simulink library "Lib_Piccolo"  (R2018b)
settings: Solver=VariableStepAuto  StartTime=0.0  StopTime=10.0  RelTol=1e-3
values from neighbouring files (symbols this model uses):
  AccelErrInt2Brakes = 0.15    [SimulationControlConfig16P.m]    (also in SimulationControlConfig16P_F0.m; SimulationControlConfig16P_F2.m; SimulationControlConfig16P_LEGACY.m; SimulationControlConfigTAILLESS.m = 0.2)
  AileronMax = 25    [SimulationControlConfig16P.m]    (also in SimulationControlConfig16P_F0.m; SimulationControlConfig16P_F2.m; SimulationControlConfig16P_LEGACY.m; SimulationControlConfigTAILLESS.m)
  AileronPower = 0.00268    [SimulationControlConfig16P.m]    (also in SimulationControlConfig16P_F0.m; SimulationControlConfig16P_F2.m; SimulationControlConfig16P_LEGACY.m; SimulationControlConfigTAILLESS.m = 0.002266)
  AileronSurfaceMax = 45    [SimulationControlConfig16P.m]    (also in SimulationControlConfig16P_F0.m; SimulationControlConfig16P_F2.m; SimulationControlConfig16P_LEGACY.m; SimulationControlConfigTAILLESS_CGAFT_F0.m = 25)
  AileronTrim = 0    [SimulationControlConfig16P.m]    (also in SimulationControlConfig16P_F0.m; SimulationControlConfig16P_F2.m; SimulationControlConfig16P_LEGACY.m; SimulationControlConfigTAILLESS.m)
  Alt = 1000 + TerrainHeight    [SimulationStateConfig.m]
  AltCruise_m = Alt * 0.3048    [SimulationControlConfig16P.m]    (also in SimulationControlConfig16P_F2.m; SimulationControlConfigTAILLESS.m = Alt/3.28084; SimulationControlConfigTAILLESS_CGAFT_F0.m = 640; SimulationControlConfigTAILLESS_CGFWD_F0.m = 640)
  AltitudeRate2PitchCmdIntegratorInit = 0.1    [SimulationControlPre.m]
  AltMax = 10000    [SimulationControlConfig16P.m]    (also in SimulationControlConfig16P_F0.m; SimulationControlConfig16P_F2.m; SimulationControlConfig16P_LEGACY.m; SimulationControlConfigTAILLESS.m)
  AltMaxAccel = 2.5    [SimulationControlConfig16P.m]    (also in SimulationControlConfig16P_F0.m = 2; SimulationControlConfig16P_F2.m = 2; SimulationControlConfig16P_LEGACY.m = 0.9; SimulationControlConfigTAILLESS.m = 2)
  AltMin = 0    [SimulationControlConfig16P.m]    (also in SimulationControlConfig16P_F0.m; SimulationControlConfig16P_F2.m; SimulationControlConfig16P_LEGACY.m; SimulationControlConfigTAILLESS.m)
  AltRateCmd2Pitch = 0.26    [SimulationControlConfig16P.m]    (also in SimulationControlConfig16P_F0.m = 0.35; SimulationControlConfig16P_F2.m = 0.35; SimulationControlConfig16P_LEGACY.m = 0.6; SimulationControlConfigTAILLESS.m = 0.9)
  AltRateError2Pitch = 0.34    [SimulationControlConfig16P.m]    (also in SimulationControlConfig16P_F0.m = 0.61; SimulationControlConfig16P_F2.m = 0.61; SimulationControlConfig16P_LEGACY.m = 0.4; SimulationControlConfigTAILLESS.m = 0.3)
  AltRateErrorInt2Pitch = 0.61    [SimulationControlConfig16P.m]    (also in SimulationControlConfig16P_F0.m = 0.28; SimulationControlConfig16P_F2.m = 0.28; SimulationControlConfig16P_LEGACY.m = 0.45; SimulationControlConfigTAILLESS.m = 0.15)
  AltRateLpfCutOff = 3    [SimulationControlConfig16P.m]    (also in SimulationControlConfig16P_F0.m; SimulationControlConfig16P_F2.m; SimulationControlConfig16P_LEGACY.m; SimulationControlConfigTAILLESS.m = 5)
  AutoNosegear2Rudder = 26    [SimulationControlConfig16P.m]    (also in SimulationControlConfig16P_F0.m; SimulationControlConfig16P_F2.m; SimulationControlConfig16P_LEGACY.m; SimulationControlConfigTAILLESS.m = 25.2)
  b = 5.54    [SimulationControlConfig16P.m]    (also in SimulationControlConfig16P_F0.m; SimulationControlConfig16P_F2.m; SimulationControlConfig16P_LEGACY.m; SimulationControlConfigTAILLESS.m = 2.37)
  Bank2AileronIntegratorInit = 0    [SimulationControlPre.m]
  BankMax_User = BankMax_User/180*pi    (= 0.610865238198)    [SimulationControlConfig16P.m]    (also in SimulationControlConfig16P_F0.m = 0.523598775598; SimulationControlConfig16P_F2.m = 0.523598775598; SimulationControlConfig16P_LEGACY.m = 0.523598775598; SimulationControlConfigTAILLESS.m = 0.558505360638)
  baseLegFlaps = 20    [SimulationControlConfig16P.m]    (also in SimulationControlConfig16P_F0.m; SimulationControlConfig16P_F2.m = 15; SimulationControlConfig16P_LEGACY.m = 0; SimulationControlConfigTAILLESS.m = 0)
  C = GeneticOpt.C    [SimulationCostFunction.m]
  c = Sw/b    (= 0.841696750903)    [SimulationControlConfig16P.m]    (also in SimulationControlConfig16P_F0.m; SimulationControlConfig16P_F2.m; SimulationControlConfig16P_LEGACY.m; SimulationControlConfigTAILLESS.m = 0.354008438819)
  cell2WheelFactorMG = 5.98    [SimulationSensorConfig16P_LEGACY.m]
  cell2WheelFactorNG = 1    [SimulationSensorConfig16P_LEGACY.m]
  cellSatMaxMG = 15000    [SimulationSensorConfig16P.m]    (also in SimulationSensorConfig16P_LEGACY.m; SimulationSensorConfigTAILLESS7P.m; SimulationSensorConfigUTAIL7P.m)
  cellSatMaxNG = 1000    [SimulationSensorConfig16P.m]    (also in SimulationSensorConfig16P_LEGACY.m; SimulationSensorConfigTAILLESS7P.m; SimulationSensorConfigUTAIL7P.m)
  cellSatMinMG = -15000    [SimulationSensorConfig16P.m]    (also in SimulationSensorConfig16P_LEGACY.m; SimulationSensorConfigTAILLESS7P.m; SimulationSensorConfigUTAIL7P.m)
  cellSatMinNG = -1000    [SimulationSensorConfig16P.m]    (also in SimulationSensorConfig16P_LEGACY.m; SimulationSensorConfigTAILLESS7P.m; SimulationSensorConfigUTAIL7P.m)
  CL_Limit = CL_Max    (= 0.54)    [SimulationControlConfig16P.m]    (also in SimulationControlConfig16P_F0.m; SimulationControlConfig16P_F2.m = 0.638; SimulationControlConfig16P_LEGACY.m; SimulationControlConfigTAILLESS.m = 0.525)
  CL_Max = 0.54    [SimulationControlConfig16P.m]    (also in SimulationControlConfig16P_F0.m; SimulationControlConfig16P_F2.m = 0.638; SimulationControlConfig16P_LEGACY.m; SimulationControlConfigTAILLESS.m = 0.525)
  CL_Max_Nom = 0.465    [SimulationControlConfig16P.m]    (also in SimulationControlConfig16P_F0.m; SimulationControlConfig16P_F2.m = 0.563; SimulationControlConfig16P_LEGACY.m; SimulationControlConfigTAILLESS.m = 0.39)
  CL_Min = 0    [SimulationControlConfig16P.m]    (also in SimulationControlConfig16P_F0.m; SimulationControlConfig16P_F2.m; SimulationControlConfig16P_LEGACY.m; SimulationControlConfigTAILLESS.m)
  ClimbMaxFraction = 0.35    [SimulationControlConfig16P.m]    (also in SimulationControlConfig16P_F0.m = 0.17; SimulationControlConfig16P_F2.m = 0.17; SimulationControlConfig16P_LEGACY.m = 0.24; SimulationControlConfigTAILLESS.m = 0.21)
  ClimboutMaxBank = 7.0    (= 7)    [SimulationControlConfig16P.m]    (also in SimulationControlConfig16P_F0.m; SimulationControlConfig16P_F2.m; SimulationControlConfig16P_LEGACY.m; SimulationControlConfigTAILLESS.m = 5)
  ClimboutTimer = 7.0    (= 7)    [SimulationControlConfig16P.m]    (also in SimulationControlConfig16P_F0.m; SimulationControlConfig16P_F2.m; SimulationControlConfig16P_LEGACY.m; SimulationControlConfigTAILLESS.m)
  dCl_per_dFlap = 0.005581818    [SimulationControlConfig16P.m]    (also in SimulationControlConfig16P_F0.m = 0; SimulationControlConfig16P_F2.m = 0.0065; SimulationControlConfig16P_LEGACY.m = 0; SimulationControlConfigTAILLESS.m = 0)
  DecelerationCmd = 3.1    [SimulationControlConfig16P.m]    (also in SimulationControlConfig16P_F0.m; SimulationControlConfig16P_F2.m; SimulationControlConfig16P_LEGACY.m; SimulationControlConfigTAILLESS.m = 0.1)
  DeRotateLogicEndTimer = abs((NoseDownLimit_Deg-1)/DeRotateRamp_Dps)    [SimulationControlConfig16P.m]    (also in SimulationControlConfig16P_F0.m; SimulationControlConfig16P_F2.m; SimulationControlConfig16P_LEGACY.m; SimulationControlConfigTAILLESS.m)
  DeRotateLogicHoldNoseUpTimer = 0.1    [SimulationControlConfig16P.m]    (also in SimulationControlConfig16P_F0.m; SimulationControlConfig16P_F2.m; SimulationControlConfig16P_LEGACY.m; SimulationControlConfigTAILLESS.m)
  DeRotateLogicTimerTimeout = 2    [SimulationControlConfig16P.m]    (also in SimulationControlConfig16P_F0.m; SimulationControlConfig16P_F2.m; SimulationControlConfig16P_LEGACY.m; SimulationControlConfigTAILLESS.m)
  DeRotateLowerCmdSaturation = 0    [SimulationControlConfig16P.m]    (also in SimulationControlConfig16P_F0.m; SimulationControlConfig16P_F2.m; SimulationControlConfig16P_LEGACY.m; SimulationControlConfigTAILLESS.m)
  DeRotateRamp_Dps = 3    [SimulationControlConfig16P.m]    (also in SimulationControlConfig16P_F0.m; SimulationControlConfig16P_F2.m; SimulationControlConfig16P_LEGACY.m; SimulationControlConfigTAILLESS.m = 8)
  DeRotateUpperCmdSaturation = 7    [SimulationControlConfig16P.m]    (also in SimulationControlConfig16P_F0.m; SimulationControlConfig16P_F2.m; SimulationControlConfig16P_LEGACY.m; SimulationControlConfigTAILLESS.m)
  DescentMaxFraction = 0.22    [SimulationControlConfig16P.m]    (also in SimulationControlConfig16P_F0.m = 0.2; SimulationControlConfig16P_F2.m = 0.2; SimulationControlConfig16P_LEGACY.m = 0.2; SimulationControlConfigTAILLESS.m = 0.17)
  DesktopSimTerrainOffset_m = 0.406    [SimulationAircraftConfig.m]
  downwindFlaps = 0    [SimulationControlConfig16P.m]    (also in SimulationControlConfig16P_F0.m; SimulationControlConfig16P_F2.m = 15; SimulationControlConfig16P_LEGACY.m; SimulationControlConfigTAILLESS.m)
  downwindSplitAil = 0    [SimulationControlConfig16P_F2.m]
  DP_init = 0.5*1.225*V_init^2    [SimulationControlConfig16P.m]    (also in SimulationControlConfig16P_F0.m; SimulationControlConfig16P_F2.m; SimulationControlConfig16P_LEGACY.m; SimulationControlConfigTAILLESS.m)
  dscNoiseMG = 1    [SimulationSensorConfig16P_LEGACY.m]
  dscNoiseNG = 0.25    [SimulationSensorConfig16P_LEGACY.m]
  DSCnumBits = 24    [SimulationSensorConfig16P.m]    (also in SimulationSensorConfig16P_LEGACY.m; SimulationSensorConfigTAILLESS7P.m; SimulationSensorConfigUTAIL7P.m)
  DSCRangeMaxMG = 15000    [SimulationSensorConfig16P.m]    (also in SimulationSensorConfig16P_LEGACY.m; SimulationSensorConfigTAILLESS7P.m; SimulationSensorConfigUTAIL7P.m)
  DSCRangeMaxNG = 1000    [SimulationSensorConfig16P.m]    (also in SimulationSensorConfig16P_LEGACY.m; SimulationSensorConfigTAILLESS7P.m; SimulationSensorConfigUTAIL7P.m)
  DSCRangeMinMG = -15000    [SimulationSensorConfig16P.m]    (also in SimulationSensorConfig16P_LEGACY.m; SimulationSensorConfigTAILLESS7P.m; SimulationSensorConfigUTAIL7P.m)
  DSCRangeMinNG = -1000    [SimulationSensorConfig16P.m]    (also in SimulationSensorConfig16P_LEGACY.m; SimulationSensorConfigTAILLESS7P.m; SimulationSensorConfigUTAIL7P.m)
  dt = DLLSim.dt    [SimulationTimeStep.m]    (also in SimulationTrim.m = 0.02)
  EarlyTouchdownThreshold = 3.0    (= 3)    [SimulationControlConfig16P.m]    (also in SimulationControlConfig16P_F0.m; SimulationControlConfig16P_F2.m; SimulationControlConfig16P_LEGACY.m; SimulationControlConfigTAILLESS.m)
  ElevatorDeflectionRate = 15    [SimulationControlConfig16P.m]    (also in SimulationControlConfig16P_F0.m; SimulationControlConfig16P_F2.m; SimulationControlConfig16P_LEGACY.m = 12; SimulationControlConfigTAILLESS.m = 5)
  ElevatorMax = 25    [SimulationControlConfig16P.m]    (also in SimulationControlConfig16P_F0.m; SimulationControlConfig16P_F2.m; SimulationControlConfig16P_LEGACY.m; SimulationControlConfigTAILLESS.m)
  ElevatorPower = -0.002209    [SimulationControlConfig16P.m]    (also in SimulationControlConfig16P_F0.m; SimulationControlConfig16P_F2.m; SimulationControlConfig16P_LEGACY.m; SimulationControlConfigTAILLESS.m = -0.002668)
  ElevatorTrim = -3.5    [SimulationControlConfig16P.m]    (also in SimulationControlConfig16P_F0.m; SimulationControlConfig16P_F2.m; SimulationControlConfig16P_LEGACY.m; SimulationControlConfigTAILLESS.m = -3)
  elevonBias = 0    [SimulationControlConfig16P.m]    (also in SimulationControlConfig16P_F0.m; SimulationControlConfig16P_F2.m; SimulationControlConfig16P_LEGACY.m; SimulationControlConfigTAILLESS.m)
  Enable_TAS_Protection = 0    [SimulationControlConfig16P.m]    (also in SimulationControlConfig16P_F0.m; SimulationControlConfig16P_F2.m; SimulationControlConfig16P_LEGACY.m; SimulationControlConfigTAILLESS.m)
  EnableCrossTrackAbort = 1    [SimulationControlConfig16P.m]    (also in SimulationControlConfigTAILLESS.m; SimulationControlConfigTAILLESS_CGAFT_F0.m; SimulationControlConfigTAILLESS_CGFWD_F0.m; SimulationControlConfigTAILLESS_CGFWD_F2.m)
  EnergyBandwidth = 0.04    [SimulationControlConfig16P.m]    (also in SimulationControlConfig16P_F0.m = 0.03; SimulationControlConfig16P_F2.m = 0.03; SimulationControlConfig16P_LEGACY.m = 0.02; SimulationControlConfigTAILLESS.m = 0.06)
  EngineLhFuelCut = 0    [SimulationAircraftConfig.m]
  EngineRhFuelCut = 0    [SimulationAircraftConfig.m]
  FastThrottleRate = 0.075    [SimulationControlConfig16P.m]    (also in SimulationControlConfig16P_F0.m = 0.05; SimulationControlConfig16P_F2.m = 0.05; SimulationControlConfig16P_LEGACY.m = 0.05; SimulationControlConfigTAILLESS.m = 0.1)
  FilterWarmUpTime = 2    [SimulationSensorConfig16P.m]    (also in SimulationSensorConfig16P_LEGACY.m; SimulationSensorConfigTAILLESS7P.m; SimulationSensorConfigUTAIL7P.m)
  finalApproachFlaps = 20    [SimulationControlConfig16P.m]    (also in SimulationControlConfig16P_F0.m; SimulationControlConfig16P_F2.m = 15; SimulationControlConfig16P_LEGACY.m = 0; SimulationControlConfigTAILLESS.m = 0)
  finalApproachSplitAil = 20    [SimulationControlConfig16P_F2.m]
  FinalDescentSlope_Deg = testPlans(testIndx).descentSlope    [SimulationControlConfig16P.m]    (also in SimulationControlConfig16P_F0.m; SimulationControlConfig16P_F2.m; SimulationControlConfig16P_LEGACY.m; SimulationControlConfigTAILLESS.m)
  flapMax = 0    [SimulationControlConfig16P.m]    (also in SimulationControlConfig16P_F0.m = 35; SimulationControlConfig16P_F2.m = 33; SimulationControlConfig16P_LEGACY.m; SimulationControlConfigTAILLESS.m)
  flapRate = 7.5    [SimulationControlConfig16P.m]    (also in SimulationControlConfig16P_F0.m; SimulationControlConfig16P_F2.m; SimulationControlConfig16P_LEGACY.m; SimulationControlConfigTAILLESS.m = 6.6)
  FlareHeight = 5    [SimulationControlConfig16P.m]    (also in SimulationControlConfig16P_F0.m; SimulationControlConfig16P_F2.m; SimulationControlConfig16P_LEGACY.m = 4.8; SimulationControlConfigTAILLESS.m = 2.75)
  FlareVerticalRate_mps = -0.4    [SimulationControlConfig16P.m]    (also in SimulationControlConfig16P_F0.m; SimulationControlConfig16P_F2.m; SimulationControlConfig16P_LEGACY.m = -0.5; SimulationControlConfigTAILLESS.m = -0.15)
  Fp_Aileron = 0.55*2*pi*RollRateLpfCutoff*dt    [SimulationControlConfig16P.m]    (also in SimulationControlConfig16P_F0.m; SimulationControlConfig16P_F2.m; SimulationControlConfig16P_LEGACY.m; SimulationControlConfigTAILLESS.m)
  Fp_Alt = 2*pi*0.55*AltBandwidth    (= 0.622035345411)    [SimulationControlConfig16P.m]    (also in SimulationControlConfig16P_F0.m; SimulationControlConfig16P_F2.m; SimulationControlConfig16P_LEGACY.m = 0.099; SimulationControlConfigTAILLESS.m = 0.207345115137)
  Fp_AltRate = 0.55*2*pi*AltRateLpfCutOff*dt    [SimulationControlConfig16P.m]    (also in SimulationControlConfig16P_F0.m; SimulationControlConfig16P_F2.m; SimulationControlConfig16P_LEGACY.m; SimulationControlConfigTAILLESS.m)
  Fp_Elevator = 0.55*2*pi*PitchRateLpfCutoff*dt    [SimulationControlConfig16P.m]    (also in SimulationControlConfig16P_F0.m; SimulationControlConfig16P_F2.m; SimulationControlConfig16P_LEGACY.m; SimulationControlConfigTAILLESS.m)
  Fp_Energy = 0.55*2*pi*EnergyBandwidth    (= 0.138230076758)    [SimulationControlConfig16P.m]    (also in SimulationControlConfig16P_F0.m = 0.103672557568; SimulationControlConfig16P_F2.m = 0.103672557568; SimulationControlConfig16P_LEGACY.m = 0.069115038379; SimulationControlConfigTAILLESS.m = 0.207345115137)
  Fp_Energy2 = 0.55*2*pi*EnergyBandwidth*dt    [SimulationControlConfig16P.m]    (also in SimulationControlConfig16P_F0.m; SimulationControlConfig16P_F2.m; SimulationControlConfig16P_LEGACY.m; SimulationControlConfigTAILLESS.m)
  Fp_Pitch = 0.55*2*pi*PitchBandwidth    (= 2.45358386245)    [SimulationControlConfig16P.m]    (also in SimulationControlConfig16P_F0.m; SimulationControlConfig16P_F2.m = 1.72787595947; SimulationControlConfig16P_LEGACY.m = 3.11017672705; SimulationControlConfigTAILLESS.m = 1.55508836353)
  Fp_Pitch_2 = 0.55*2*pi*PitchBandwidth*dt    [SimulationControlConfig16P.m]    (also in SimulationControlConfig16P_F0.m; SimulationControlConfig16P_F2.m; SimulationControlConfig16P_LEGACY.m; SimulationControlConfigTAILLESS.m)
  Fp_Roll = RollBandwidth^2    (= 1.69)    [SimulationControlConfig16P.m]    (also in SimulationControlConfig16P_F0.m = 1.44; SimulationControlConfig16P_F2.m = 1.44; SimulationControlConfig16P_LEGACY.m = 1.44; SimulationControlConfigTAILLESS.m = 1.21)
  Fp_Rudder = 0.55*2*pi*YawRateLpfCutoff*dt    [SimulationControlConfig16P.m]    (also in SimulationControlConfig16P_F0.m; SimulationControlConfig16P_F2.m; SimulationControlConfig16P_LEGACY.m; SimulationControlConfigTAILLESS.m)
  Fp_TAS = 0.55*2*pi*TASBandwidth    (= 0.103672557568)    [SimulationControlConfig16P.m]    (also in SimulationControlConfig16P_F0.m; SimulationControlConfig16P_F2.m; SimulationControlConfig16P_LEGACY.m; SimulationControlConfigTAILLESS.m = 0.172787595947)
  Fp_TAS_Filter = 2*pi*TasLpfCutoff*dt    [SimulationControlConfig16P.m]    (also in SimulationControlConfig16P_F0.m; SimulationControlConfig16P_F2.m; SimulationControlConfig16P_LEGACY.m; SimulationControlConfigTAILLESS.m)
  Fp_Turn = 0.55*2*pi*TurnErrLPFcutoff    (= 0.172787595947)    [SimulationControlConfig16P.m]    (also in SimulationControlConfig16P_F0.m = 0.0345575191895; SimulationControlConfig16P_F2.m = 0.0345575191895; SimulationControlConfig16P_LEGACY.m = 0.0345575191895; SimulationControlConfigTAILLESS.m)
  Fp_TurnDerr = 0.55*2*pi*TurnDerivativeLPFcutoff    (= 0.172787595947)    [SimulationControlConfig16P.m]    (also in SimulationControlConfig16P_F0.m = 0.0345575191895; SimulationControlConfig16P_F2.m = 0.0345575191895; SimulationControlConfig16P_LEGACY.m = 0.0345575191895; SimulationControlConfigTAILLESS.m)
  FTV = 3    [SimulationAircraftConfig.m]
  ftvStaticPositionError = 1/1.18    (= 0.847457627119)    [SimulationSensorConfig16P.m]    (also in SimulationSensorConfig16P_LEGACY.m; SimulationSensorConfigTAILLESS7P.m = 1; SimulationSensorConfigUTAIL7P.m = 1)
  g = 9.81    [SimulationStateConfig.m]
  goAroundSplitAil = 0    [SimulationControlConfig16P_F2.m]
  GustSpd_Kts = testPlans(testIndx).gustSpd    [SimulationStateConfig.m]
  GustTriggerVal = testPlans(testIndx).gustTriggerVal    [SimulationStateConfig.m]
  HeadingErr2TurnRate = 0.5    [SimulationControlConfig16P.m]    (also in SimulationControlConfig16P_F0.m; SimulationControlConfig16P_F2.m; SimulationControlConfig16P_LEGACY.m; SimulationControlConfigTAILLESS.m)
  HeadingErrDer2TurnRate = 0.3    [SimulationControlConfig16P.m]    (also in SimulationControlConfig16P_F0.m; SimulationControlConfig16P_F2.m; SimulationControlConfig16P_LEGACY.m; SimulationControlConfigTAILLESS.m)
  IASbounce = IASstall*0.8    [SimulationControlPre.m]
  IAScruiseCMD = sqrt(2*m*9.81/(1.225*Sw*CL_cruise))    [SimulationControlConfig16P.m]    (also in SimulationControlConfig16P_F0.m; SimulationControlConfig16P_F2.m; SimulationControlConfig16P_LEGACY.m; SimulationControlConfigTAILLESS.m)
  IASfinalCMD = 1.12 * IASmin    [SimulationControlConfig16P.m]    (also in SimulationControlConfig16P_F0.m = 1.14 * IASmin; SimulationControlConfig16P_F2.m = 1.10 * IASmin; SimulationControlConfig16P_LEGACY.m = 1.10 * IASmin; SimulationControlConfigTAILLESS.m = 1.14 * IASmin)
  IASflareCMD = IASstall    [SimulationControlConfig16P.m]    (also in SimulationControlConfig16P_F0.m; SimulationControlConfig16P_F2.m; SimulationControlConfig16P_LEGACY.m; SimulationControlConfigTAILLESS.m)
  IASmax = 64    [SimulationControlConfig16P.m]    (also in SimulationControlConfig16P_F0.m = 46; SimulationControlConfig16P_F2.m = 52; SimulationControlConfig16P_LEGACY.m = 46; SimulationControlConfigTAILLESS.m = 38.9)
  IASmin = sqrt(2*m*9.81/(1.225*Sw*0.9*CL_Max_Nom))    [SimulationControlConfig16P.m]    (also in SimulationControlConfig16P_F0.m; SimulationControlConfig16P_F2.m; SimulationControlConfig16P_LEGACY.m; SimulationControlConfigTAILLESS.m)
  IASshortCMD = IASstall    [SimulationControlConfig16P.m]    (also in SimulationControlConfig16P_F0.m; SimulationControlConfig16P_F2.m; SimulationControlConfig16P_LEGACY.m; SimulationControlConfigTAILLESS.m)
  IASstall = sqrt(2*m*9.81/(1.225*Sw*CL_Max))    [SimulationControlConfig16P.m]    (also in SimulationControlConfig16P_F0.m; SimulationControlConfig16P_F2.m; SimulationControlConfig16P_LEGACY.m; SimulationControlConfigTAILLESS.m)
  inFlight = 1    [SimulationControlConfig16P.m]    (also in SimulationControlConfigTAILLESS.m; SimulationControlConfigTAILLESS_CGAFT_F0.m; SimulationControlConfigTAILLESS_CGFWD_F0.m; SimulationControlConfigTAILLESS_CGFWD_F2.m)
  JetCatOffset = 5    [SimulationControlConfig16P.m]    (also in SimulationControlConfig16P_F0.m; SimulationControlConfig16P_F2.m; SimulationControlConfig16P_LEGACY.m)
  LaunchRollingElevator = -1.5    [SimulationControlConfig16P.m]    (also in SimulationControlConfig16P_F0.m; SimulationControlConfig16P_F2.m = 1.25; SimulationControlConfig16P_LEGACY.m; SimulationControlConfigTAILLESS.m = 1)
  ldg_NosegearMax = 10    [SimulationControlConfig16P.m]    (also in SimulationControlConfig16P_F0.m; SimulationControlConfig16P_F2.m; SimulationControlConfig16P_LEGACY.m; SimulationControlConfigTAILLESS.m)
  ldg_TrackVyErrInt2Nosegear = 0.1250    (= 0.125)    [SimulationControlConfig16P.m]    (also in SimulationControlConfig16P_F0.m; SimulationControlConfig16P_F2.m; SimulationControlConfig16P_LEGACY.m; SimulationControlConfigTAILLESS.m = 0.00714285714286)
  ldg_TrackVyErrPro2Nosegear = 0.35    [SimulationControlConfig16P.m]    (also in SimulationControlConfig16P_F0.m; SimulationControlConfig16P_F2.m; SimulationControlConfig16P_LEGACY.m; SimulationControlConfigTAILLESS.m = 0.0546666666667)
  ldg_TrackY2Vy = 0.07    [SimulationControlConfig16P.m]    (also in SimulationControlConfig16P_F0.m; SimulationControlConfig16P_F2.m; SimulationControlConfig16P_LEGACY.m; SimulationControlConfigTAILLESS.m = 0.17)
  ldg_Vy2NosegearScalingPower = 1.075    [SimulationControlConfig16P.m]    (also in SimulationControlConfig16P_F0.m; SimulationControlConfig16P_F2.m; SimulationControlConfig16P_LEGACY.m; SimulationControlConfigTAILLESS.m = 0.6)
  ldg_Y2VyScalingPower = 0.175    [SimulationControlConfig16P.m]    (also in SimulationControlConfig16P_F0.m; SimulationControlConfig16P_F2.m; SimulationControlConfig16P_LEGACY.m; SimulationControlConfigTAILLESS.m = 0)
  ldg_YawRate2Nosegear = 0.175    [SimulationControlConfig16P.m]    (also in SimulationControlConfig16P_F0.m; SimulationControlConfig16P_F2.m; SimulationControlConfig16P_LEGACY.m; SimulationControlConfigTAILLESS.m = 0.065)
  LiftSlope = 0.064285    [SimulationControlConfig16P.m]    (also in SimulationControlConfig16P_F0.m; SimulationControlConfig16P_F2.m; SimulationControlConfig16P_LEGACY.m; SimulationControlConfigTAILLESS.m = 0.058631)
  LPFaileronInit = 0    [SimulationControlPre.m]
  LPFclestInit = 0    [SimulationControlPre.m]
  LPFenergyFFInit = 0    [SimulationControlPre.m]
  ... (+122 more)
undefined symbols (not defined in the file or in its folder): abortFlag, alphaHPF, apmDelay, BRWNOUT, CRAWOR, CRAWUR, DiscIntNeverNeededParam, DLLSim, DLLSimStep, ECOMOR, ECOMUR, Fp_Tas, GustTrigger_HeightAgl_m, IPSTAT, LCINTEG, Ldg_Persist_Time, LOWER_FLAGS, MSG_ENABLE, NoiseStd, OLDVAL, OVERRIDE_ENABLE, OVERRIDE_VALUE, REBOOT, reversionEnable, revIASMax, revIASMin, revPitchMax, revPitchMin, revPitchRateMax, revRollMax, revRollRateMax, SAMPLE, SCALON, SensorModel, sigbuilder_block, Sim_Vx, Sim_Vy, Sim_Vz, Sim_Xpos, Sim_Ypos, Sim_Zpos, SYSOR, SYSUR, TARE, TEMPOR, TEMPUR, testIndx, testPlan, testPlans, Trim_piccoloInCmd, Trim_REFSI_FD_IN_nmodeCgShifterCmd_Flag, Trim_REFSI_FD_IN_nmodeCgShifterCmd_Ft, Trim_REFSI_FD_IN_nmodeCgShifterCmdType, Trim_REFSI_FD_IN_nmodeCgShifterNRCActive, Trim_REFSI_FD_IN_nmodeFlapLhIBCmd_Deg, Trim_REFSI_FD_IN_nmodeFlapLhOBCmd_Deg, Trim_REFSI_FD_IN_nmodeFlapRhIBCmd_Deg, Trim_REFSI_FD_IN_nmodeFlapRhOBCmd_Deg, Trim_REFSI_FD_IN_nmodeSlatLhCmd_Deg ... (+11)
libraries: simulink x1237, $bdroot x179, aerolibconvert2 x63, dspswit3 x25, aerolibatmos2 x5, simulink_extras x4, dsparch4 x2, Lib_Piccolo_Alt x2, eeGeneralControl x1, dspindex x1
(part 54 of 74)

== system Lib_Piccolo/Ground Detection Systems/WoW Wrapper/Variant Subsystem/Load Cell WoW Model 20/WOW Module/T//O Configuration ==
  note: Unlike when landing our persistance and latching is inverted relative to Weight Off both gears.
      |
      | Protection against WOW Failure. In the Event of a Sensor Failure and AC lift's off, NZ threshold overides WOW signal.
  WOW_Filt : Inport
  DSC_Fail : Inport  Port=2
  AND : Logic  IconShape=distinctive  AllPortsSameDT=off  OutDataTypeStr=boolean
  Bus Selector : BusSelector  OutputSignals=WOW_Filt_NG_N,WOW_Filt_MGL_N,WOW_Filt_MGR_N
  Bus Selector1 : BusSelector  OutputSignals=MGR_DSC_FAIL,MGL_DSC_FAIL
  Compare To Constant1 : simulink/Logic and Bit Operations/Compare To Constant  relop=<  const=SensorModel.WOW.Cell.TO_loadThreshold_N  OutDataTypeStr=uint8
  Compare To Constant2 : simulink/Logic and Bit Operations/Compare To Constant  relop=<  const=SensorModel.WOW.Cell.TO_loadThreshold_N  OutDataTypeStr=uint8
  Input Selection (Failure Handling) : $bdroot/Ground Detection Systems/WoW Wrapper/Variant Subsystem/Load Cell WoW Model 20/WOW Module/Landing Configuration/Input Selection (Failure Handling)  SystemSampleTime=-1
  Latch : Subsystem
  Latch Timer : Subsystem  mask{period=SensorModel.WOW.Cell.TO_latchTime_s}
      mask prompts: period "Period [s]"
  NOT : Logic  Operator=NOT  IconShape=distinctive  AllPortsSameDT=off  OutDataTypeStr=boolean
  NOT2 : Logic  Operator=NOT  IconShape=distinctive  AllPortsSameDT=off  OutDataTypeStr=boolean
  Persistance Timer : Subsystem  mask{period=SensorModel.WOW.Cell.TO_persistanceTime_s}
      mask prompts: period "Period [s]"
  Terminator : Terminator
  Unit Delay : UnitDelay  SampleTime=-1
  ContactBool : Outport
  Takeoff_Fail_L : Outport  Port=2
  Takeoff_Fail_R : Outport  Port=3
  wires:
  NOT2/1 -> ContactBool/1
  Persistance Timer/1(Expired) -> Latch/1(D)
  Compare To Constant2/1 -> AND/1
  Latch Timer/1(Expired) -> NOT/1
  Unit Delay/1 -> Latch Timer/1(Enable/!Rst)
  Compare To Constant1/1 -> AND/2
  AND/1 -> Persistance Timer/1(Enable/!Rst)
  Latch/1(Q_Latched) -> NOT2/1, Unit Delay/1  "ContactBool"
  NOT/1 -> Latch/2(Enable/!Rst)
  WOW_Filt/1 -> Bus Selector/1
  Bus Selector/1 -> Terminator/1  "<WOW_Filt_NG_N>"
  Bus Selector/2 -> Input Selection (Failure Handling)/1  "<WOW_Filt_MGL_N>"
  Bus Selector/3 -> Input Selection (Failure Handling)/2  "<WOW_Filt_MGR_N>"
  DSC_Fail/1 -> Bus Selector1/1
  Bus Selector1/1 -> Input Selection (Failure Handling)/3  "<MGR_DSC_FAIL>"
  Bus Selector1/2 -> Input Selection (Failure Handling)/4  "<MGL_DSC_FAIL>"
  Input Selection (Failure Handling)/1 -> Compare To Constant2/1  "InputL"
  Input Selection (Failure Handling)/2 -> Compare To Constant1/1  "InputR"
  Input Selection (Failure Handling)/3 -> Takeoff_Fail_L/1
  Input Selection (Failure Handling)/4 -> Takeoff_Fail_R/1

== system Lib_Piccolo/Ground Detection Systems/WoW Wrapper/Variant Subsystem/Load Cell WoW Model 20/WOW Module/Tare ==
  note: Use DSC health information to select tare value.
      |
      | If DSC is failed, use previous tare value (don't update).
      |
      | Else, sample LPF for that channel and update tare value.
  WOW_Bias_Filt_N : Inport
  DSC_Fail : Inport  Port=2
  Tare_In : Inport  Port=3
  Trigger : TriggerPort  VariantControl=Variant  PortDimensions=1
  Bus Selector : BusSelector  OutputSignals=Bias_NG_N,Bias_MGL_N,Bias_MGR_N
  Bus Selector1 : BusSelector  OutputSignals=NG_DSC_FAIL,MGL_DSC_FAIL,MGR_DSC_FAIL
  Bus Selector2 : BusSelector  OutputSignals=NG_TARE_N,MGL_TARE_N,MGR_TARE_N
  Switch : Switch  Criteria=u2 > Threshold  Threshold=0.5
  Switch1 : Switch  Criteria=u2 > Threshold  Threshold=0.5
  Switch2 : Switch  Criteria=u2 > Threshold  Threshold=0.5
  NG_TARE_N : Outport  OutDataTypeStr=single
  MGL_TARE_N : Outport  Port=2  OutDataTypeStr=single
  MGR_TARE_N : Outport  Port=3  OutDataTypeStr=single
  wires:
  WOW_Bias_Filt_N/1 -> Bus Selector/1
  Bus Selector/1 -> [Bias_NG_N]  "<Bias_NG_N>"
  Bus Selector/2 -> [Bias_MGL_N]  "<Bias_MGL_N>"
  Bus Selector/3 -> [Bias_MGR_N]  "<Bias_MGR_N>"
  DSC_Fail/1 -> Bus Selector1/1
  Bus Selector1/3 -> Switch2/2  "<MGR_DSC_FAIL>"
  Bus Selector1/2 -> Switch1/2  "<MGL_DSC_FAIL>"
  Bus Selector1/1 -> Switch/2  "<NG_DSC_FAIL>"
  Tare_In/1 -> Bus Selector2/1
  Bus Selector2/1 -> [NG_TARE]  "<NG_TARE_N>"
  Bus Selector2/2 -> [MGL_TARE]  "<MGL_TARE_N>"
  Bus Selector2/3 -> [MGR_TARE]  "<MGR_TARE_N>"
  [NG_TARE] -> Switch/1
  Switch/1 -> NG_TARE_N/1
  [Bias_NG_N] -> Switch/3
  Switch1/1 -> MGL_TARE_N/1
  [Bias_MGL_N] -> Switch1/3
  [MGL_TARE] -> Switch1/1
  [MGR_TARE] -> Switch2/1
  [Bias_MGR_N] -> Switch2/3
  Switch2/1 -> MGR_TARE_N/1

== system Lib_Piccolo/Ground Detection Systems/WoW Wrapper/Variant Subsystem/Load Cell WoW Model 21/Load Cell and Unit Conversion/Conversion - MGL ==
  Lbf : Inport
  Lbf2N : Gain  Gain=4.44822
  N : Outport
  wires:
  Lbf/1 -> Lbf2N/1
  Lbf2N/1 -> N/1

== system Lib_Piccolo/Ground Detection Systems/WoW Wrapper/Variant Subsystem/Load Cell WoW Model 21/Load Cell and Unit Conversion/Conversion - MGR ==
  Lbf : Inport
  Lbf2N : Gain  Gain=4.44822
  N : Outport
  wires:
  Lbf/1 -> Lbf2N/1
  Lbf2N/1 -> N/1

== system Lib_Piccolo/Ground Detection Systems/WoW Wrapper/Variant Subsystem/Load Cell WoW Model 21/Load Cell and Unit Conversion/Conversion - NG ==
  Lbf : Inport
  Lbf2N : Gain  Gain=4.44822
  N : Outport
  wires:
  Lbf2N/1 -> N/1
  Lbf/1 -> Lbf2N/1

== system Lib_Piccolo/Ground Detection Systems/WoW Wrapper/Variant Subsystem/Load Cell WoW Model 21/Load Cell and Unit Conversion/Wheel-to-Cell Scaling MGL ==
  Wheel Load N : Inport
  Square : Math  Operator=square  SaturateOnIntegerOverflow=on
  Sum : Sum  Inputs=+++
  a : Gain  Gain=polyA
  b : Gain  Gain=polyB
  c : Constant  Value=polyC
  Cell Load N : Outport  VectorParamsAs1DForOutWhenUnconnected=on
  wires:
  Wheel Load N/1 -> b/1, Square/1
  Square/1 -> a/1
  b/1 -> Sum/2
  a/1 -> Sum/1
  c/1 -> Sum/3
  Sum/1 -> Cell Load N/1

== system Lib_Piccolo/Ground Detection Systems/WoW Wrapper/Variant Subsystem/Load Cell WoW Model 21/Load Cell and Unit Conversion/Wheel-to-Cell Scaling MGR ==
  Wheel Load N : Inport
  Square : Math  Operator=square  SaturateOnIntegerOverflow=on
  Sum : Sum  Inputs=+++
  a : Gain  Gain=polyA
  b : Gain  Gain=polyB
  c : Constant  Value=polyC
  Cell Load N : Outport  VectorParamsAs1DForOutWhenUnconnected=on
  wires:
  Wheel Load N/1 -> b/1, Square/1
  Square/1 -> a/1
  b/1 -> Sum/2
  a/1 -> Sum/1
  c/1 -> Sum/3
  Sum/1 -> Cell Load N/1

== system Lib_Piccolo/Ground Detection Systems/WoW Wrapper/Variant Subsystem/Load Cell WoW Model 21/Load Cell and Unit Conversion/Wheel-to-Cell Scaling NG ==
  Wheel Load N : Inport
  Square : Math  Operator=square  SaturateOnIntegerOverflow=on
  Sum : Sum  Inputs=+++
  a : Gain  Gain=polyA
  b : Gain  Gain=polyB
  c : Constant  Value=polyC
  Cell Load N : Outport  VectorParamsAs1DForOutWhenUnconnected=on
  wires:
  Wheel Load N/1 -> b/1, Square/1
  Square/1 -> a/1
  b/1 -> Sum/2
  a/1 -> Sum/1
  c/1 -> Sum/3
  Sum/1 -> Cell Load N/1

== system Lib_Piccolo/Ground Detection Systems/WoW Wrapper/Variant Subsystem/Load Cell WoW Model 21/WOW Module/Bias Filters ==
  WOW_NG_RAW_N : Inport
  WOW_MGL_RAW_N : Inport  Port=2
  WOW_MGR_RAW_N : Inport  Port=3
  Bus Creator : BusCreator  Inputs=3
  Ground : Ground
  LPF MGL : Subsystem  mask{Cutoff=SensorModel.WOW.Cell.fc, Init=0}
      mask prompts: Cutoff "Cutoff Frequency [Hz]"; Init "Initial Condition"
  LPF MGR : Subsystem  mask{Cutoff=SensorModel.WOW.Cell.fc, Init=0}
      mask prompts: Cutoff "Cutoff Frequency [Hz]"; Init "Initial Condition"
  LPF NG : Subsystem  mask{Cutoff=SensorModel.WOW.Cell.fc, Init=0}
      mask prompts: Cutoff "Cutoff Frequency [Hz]"; Init "Initial Condition"
  WOW_Bias_Filt_N : Outport  VectorParamsAs1DForOutWhenUnconnected=on
  wires:
  WOW_NG_RAW_N/1 -> LPF NG/1("Input ")
  Bus Creator/1 -> WOW_Bias_Filt_N/1
  LPF NG/1("Output ") -> Bus Creator/1  "Bias_NG_N"
  Ground/1 -> LPF MGL/2(Reset), LPF MGR/2(Reset), LPF NG/2(Reset)
  WOW_MGL_RAW_N/1 -> LPF MGL/1("Input ")
  LPF MGL/1("Output ") -> Bus Creator/2  "Bias_MGL_N"
  LPF MGR/1("Output ") -> Bus Creator/3  "Bias_MGR_N"
  WOW_MGR_RAW_N/1 -> LPF MGR/1("Input ")

== system Lib_Piccolo/Ground Detection Systems/WoW Wrapper/Variant Subsystem/Load Cell WoW Model 21/WOW Module/Command Processing ==
  User Cmd Bus In : Inport
  Bus Selector : BusSelector  OutputSignals=MSG_ENABLE,TARE,OVERRIDE_ENABLE,OVERRIDE_VALUE
  Edge Detector : dspswit3/Edge Detector  InputProcessing=Columns as channels (frame based)
      settings: SourceProductName=DSP System Toolbox  SourceProductBaseCode=DS
  TARE_TRIGGER : Outport
  MSG_ENABLE : Outport  Port=2
  OVERRIDE_ENABLE : Outport  Port=3  OutDataTypeStr=boolean  VectorParamsAs1DForOutWhenUnconnected=on
  OVERRIDE_VALUE : Outport  Port=4  OutDataTypeStr=boolean  VectorParamsAs1DForOutWhenUnconnected=on
  User Cmd Bus Out : Outport  Port=5
  wires:
  Bus Selector/1 -> MSG_ENABLE/1  "<MSG_ENABLE>"
  User Cmd Bus In/1 -> Bus Selector/1, User Cmd Bus Out/1
  Bus Selector/2 -> Edge Detector/1  "<TARE>"
  Edge Detector/1 -> TARE_TRIGGER/1
  Bus Selector/3 -> OVERRIDE_ENABLE/1  "<OVERRIDE_ENABLE>"
  Bus Selector/4 -> OVERRIDE_VALUE/1  "<OVERRIDE_VALUE>"

== system Lib_Piccolo/Ground Detection Systems/WoW Wrapper/Variant Subsystem/Load Cell WoW Model 21/WOW Module/Flag Latch ==
  note: Latch failure/disable state if AP mode is <= climbout, or >= final
  INIT : Inport
  OUTPUT_DISABLE : Inport  Port=2
  PIC_AP_MODE : Inport  Port=3
  Latch : Subsystem
  Latch Activation on Mode : Subsystem
  OR5 : Logic  Operator=OR  IconShape=distinctive  AllPortsSameDT=off  OutDataTypeStr=boolean
  OUTPUT_DISABLE_LATCHED : Outport
  wires:
  INIT/1 -> OR5/1
  Latch/1(Q_Latched) -> OUTPUT_DISABLE_LATCHED/1
  OUTPUT_DISABLE/1 -> OR5/2
  OR5/1 -> Latch/1(D)
  PIC_AP_MODE/1 -> Latch Activation on Mode/1(Piccolo Mode)
  Latch Activation on Mode/1(Mode Latch) -> Latch/2(Enable/!Rst)

== system Lib_Piccolo/Ground Detection Systems/WoW Wrapper/Variant Subsystem/Load Cell WoW Model 21/WOW Module/LPF MGL ==
  "Input " : Inport
  Reset : Inport  Port=2
  Add1 : Sum  Inputs=++|
  Compare To Constant2 : simulink/Logic and Bit Operations/Compare To Constant  relop=>  const=0  OutDataTypeStr=uint8
  Constant11 : Constant  Value=Cutoff
  Resettable Delay : Delay  DelayLength=1  InitialConditionSource=Input port  ExternalReset=Level hold
      settings: InputPortMap=u0,r5,p4
  Switch1 : Switch  Criteria=u2 > Threshold
  a1 : Gain  Gain=SensorModel.WOW.Cell.a1
  b0 : Gain  Gain=SensorModel.WOW.Cell.b0
  "Output " : Outport
  wires:
  Resettable Delay/1 -> a1/1
  b0/1 -> Add1/2
  Add1/1 -> Resettable Delay/1, Switch1/1
  a1/1 -> Add1/1
  "Input "/1 -> b0/1, Switch1/3, Resettable Delay/3
  Switch1/1 -> "Output "/1
  Compare To Constant2/1 -> Switch1/2
  Constant11/1 -> Compare To Constant2/1
  Reset/1 -> Resettable Delay/2

== system Lib_Piccolo/Ground Detection Systems/WoW Wrapper/Variant Subsystem/Load Cell WoW Model 21/WOW Module/LPF MGR ==
  "Input " : Inport
  Reset : Inport  Port=2
  Add1 : Sum  Inputs=++|
  Compare To Constant2 : simulink/Logic and Bit Operations/Compare To Constant  relop=>  const=0  OutDataTypeStr=uint8
  Constant11 : Constant  Value=Cutoff
  Resettable Delay : Delay  DelayLength=1  InitialConditionSource=Input port  ExternalReset=Level hold
      settings: InputPortMap=u0,r5,p4
  Switch1 : Switch  Criteria=u2 > Threshold
  a1 : Gain  Gain=SensorModel.WOW.Cell.a1
  b0 : Gain  Gain=SensorModel.WOW.Cell.b0
  "Output " : Outport
  wires:
  Resettable Delay/1 -> a1/1
  b0/1 -> Add1/2
  Add1/1 -> Resettable Delay/1, Switch1/1
  a1/1 -> Add1/1
  "Input "/1 -> b0/1, Switch1/3, Resettable Delay/3
  Switch1/1 -> "Output "/1
  Compare To Constant2/1 -> Switch1/2
  Constant11/1 -> Compare To Constant2/1
  Reset/1 -> Resettable Delay/2

== system Lib_Piccolo/Ground Detection Systems/WoW Wrapper/Variant Subsystem/Load Cell WoW Model 21/WOW Module/LPF NG ==
  "Input " : Inport
  Reset : Inport  Port=2
  Add1 : Sum  Inputs=++|
  Compare To Constant2 : simulink/Logic and Bit Operations/Compare To Constant  relop=>  const=0  OutDataTypeStr=uint8
  Constant11 : Constant  Value=Cutoff
  Resettable Delay : Delay  DelayLength=1  InitialConditionSource=Input port  ExternalReset=Level hold
      settings: InputPortMap=u0,r5,p4
  Switch1 : Switch  Criteria=u2 > Threshold
  a1 : Gain  Gain=SensorModel.WOW.Cell.a1
  b0 : Gain  Gain=SensorModel.WOW.Cell.b0
  "Output " : Outport
  wires:
  Reset/1 -> Resettable Delay/2
  Constant11/1 -> Compare To Constant2/1
  Compare To Constant2/1 -> Switch1/2
  Switch1/1 -> "Output "/1
  "Input "/1 -> b0/1, Switch1/3, Resettable Delay/3
  a1/1 -> Add1/1
  Add1/1 -> Switch1/1, Resettable Delay/1
  b0/1 -> Add1/2
  Resettable Delay/1 -> a1/1

== system Lib_Piccolo/Ground Detection Systems/WoW Wrapper/Variant Subsystem/Load Cell WoW Model 21/WOW Module/Landing Configuration ==
  WOW_Filt : Inport
  DSC_Fail : Inport  Port=2
  PICCOLO_AP_MODE : Inport  Port=3
  AND1 : Logic  IconShape=distinctive  AllPortsSameDT=off  OutDataTypeStr=boolean
  Bus Selector : BusSelector  OutputSignals=WOW_Filt_NG_N,WOW_Filt_MGL_N,WOW_Filt_MGR_N
  Bus Selector1 : BusSelector  OutputSignals=MGR_DSC_FAIL,MGL_DSC_FAIL
  Enable : Constant  Value=SensorModel.WOW.Cell.useDualLogic
  Gain1 : Gain
  Gain2 : Gain
  Hysteresis L : Relay  OnSwitchValue=SensorModel.WOW.Cell.loadThresholdUpper_N  OffSwitchValue=SensorModel.WOW.Cell.loadThresholdLower_N
  Hysteresis R : Relay  OnSwitchValue=SensorModel.WOW.Cell.loadThresholdUpper_N  OffSwitchValue=SensorModel.WOW.Cell.loadThresholdLower_N
  Input Selection (Failure Handling) : Subsystem
  Latching Logic : Subsystem
  Logic Selection : Subsystem
  Persistance Timer : Subsystem  mask{period=SensorModel.WOW.Cell.persistanceTime_s}
      mask prompts: period "Period [s]"
  Terminator{,1..3} (4 alike) : Terminator
  Timeout Logic : Subsystem
  Unit Delay : UnitDelay  SampleTime=-1
  ContactBool : Outport
  Landing_Fail_L : Outport  Port=2
  Landing_Fail_R : Outport  Port=3
  wires:
  Enable/1 -> AND1/1
  AND1/1 -> Logic Selection/2(Logic Mode (Or/!And)), Timeout Logic/2(Logic Mode (Or/!And))  "Logic Mode (Or/!And)"
  [Contact] -> AND1/2
  Bus Selector/1 -> Terminator/1  "<WOW_Filt_NG_N>"
  WOW_Filt/1 -> Bus Selector/1
  Gain2/1 -> Terminator2/1  "ContactR"
  Gain1/1 -> Terminator1/1  "ContactL"
  Hysteresis R/1 -> Gain2/1, Logic Selection/3(ContactR), Timeout Logic/3(ContactR)
  Hysteresis L/1 -> Timeout Logic/1(ContactL), Logic Selection/1(ContactL), Gain1/1
  Unit Delay/1 -> [Contact]
  Latching Logic/1(ContactOut) -> ContactBool/1, Unit Delay/1  "ContactBool"
  DSC_Fail/1 -> Bus Selector1/1
  Input Selection (Failure Handling)/2(InputR) -> Hysteresis R/1  "InputR"
  Input Selection (Failure Handling)/1(InputL) -> Hysteresis L/1  "InputL"
  Persistance Timer/1(Expired) -> Latching Logic/1(ContactIn)
  Bus Selector/2 -> Input Selection (Failure Handling)/1(WOW_Filt_MGL_N)  "<WOW_Filt_MGL_N>"
  Bus Selector/3 -> Input Selection (Failure Handling)/2(WOW_Filt_MGR_N)  "<WOW_Filt_MGR_N>"
  Bus Selector1/1 -> Input Selection (Failure Handling)/3(MGR_DSC_FAIL)  "<MGR_DSC_FAIL>"
  Bus Selector1/2 -> Input Selection (Failure Handling)/4(MGL_DSC_FAIL)  "<MGL_DSC_FAIL>"
  Logic Selection/1(ContactOut) -> Persistance Timer/1(Enable/!Rst)
  Input Selection (Failure Handling)/4(FailR) -> Landing_Fail_R/1
  Input Selection (Failure Handling)/3(FailL) -> Landing_Fail_L/1
  PICCOLO_AP_MODE/1 -> Terminator3/1

== system Lib_Piccolo/Ground Detection Systems/WoW Wrapper/Variant Subsystem/Load Cell WoW Model 21/WOW Module/Override Logic ==
  Logic Contact : Inport
  Override Enable : Inport  Port=2
  Override Value : Inport  Port=3
  Constant : Constant  Value=100  OutDataTypeStr=uint8
  Constant1 : Constant  Value=0  OutDataTypeStr=uint8
  Switch : Switch  Criteria=u2 > Threshold  Threshold=0.5
  Switch1 : Switch  Criteria=u2 > Threshold  Threshold=0.5
  CONTACT : Outport  VectorParamsAs1DForOutWhenUnconnected=on
  WOW_PCNT : Outport  Port=2  OutDataTypeStr=uint8  VectorParamsAs1DForOutWhenUnconnected=on
  wires:
  Override Enable/1 -> Switch/2
  Switch/1 -> Switch1/2, CONTACT/1
  Override Value/1 -> Switch/1
  Logic Contact/1 -> Switch/3
  Switch1/1 -> WOW_PCNT/1
  Constant/1 -> Switch1/1
  Constant1/1 -> Switch1/3

== system Lib_Piccolo/Ground Detection Systems/WoW Wrapper/Variant Subsystem/Load Cell WoW Model 21/WOW Module/Subsystem ==
  WOW_Bus : Inport
  MGR FLAG Word : Inport  Port=2
  MGR STAT Word : Inport  Port=3
  MGL FLAG Word : Inport  Port=4
  MGL STAT Word : Inport  Port=5
  NG FLAG Word : Inport  Port=6
  NG STAT Word : Inport  Port=7
  MGR_STALE_LOAD : Inport  Port=8  OutDataTypeStr=boolean
  MGR_STALE_FLAGS : Inport  Port=9  OutDataTypeStr=boolean
  MGL_STALE_LOAD : Inport  Port=10  OutDataTypeStr=boolean
  MGL_STALE_FLAGS : Inport  Port=11  OutDataTypeStr=boolean
  NG_STALE_LOAD : Inport  Port=12  OutDataTypeStr=boolean
  NG_STALE_FLAGS : Inport  Port=13  OutDataTypeStr=boolean
  NRC Active : Inport  Port=14
  PIC_AP_MODE : Inport  Port=15  OutDataTypeStr=uint8
  INIT : Inport  Port=16
  " Output Formatting" : Subsystem
  AND : Logic  Inputs=3  IconShape=distinctive  AllPortsSameDT=off  OutDataTypeStr=boolean
  AND1 : Logic  IconShape=distinctive  AllPortsSameDT=off
  AND2 : Logic  Inputs=3  IconShape=distinctive  AllPortsSameDT=off  OutDataTypeStr=boolean
  AND3 : Logic  Inputs=3  IconShape=distinctive  AllPortsSameDT=off  OutDataTypeStr=boolean
  Bus Assignment : BusAssignment  AssignedSignals=ACTIVE
  Bus Assignment1 : BusAssignment  AssignedSignals=ACTIVE
  Bus Assignment2 : BusAssignment  AssignedSignals=ACTIVE
  Bus Selector : BusSelector  OutputSignals=WOW_MGR_Filt_N,WOW_MGL_Filt_N,WOW_NG_Filt_N
  Comms Timeout Logic : Subsystem
  Health Check : Subsystem
  NOT : Logic  Operator=NOT  IconShape=distinctive  AllPortsSameDT=off  OutDataTypeStr=boolean
  MGR_DSC_FAIL : Outport  OutDataTypeStr=boolean
  MGL_DSC_FAIL : Outport  Port=2  OutDataTypeStr=boolean
  NG_DSC_FAIL : Outport  Port=3  OutDataTypeStr=boolean
  OUTPUT_DISABLE : Outport  Port=4
  NG_Out : Outport  Port=5
  MGL_Out : Outport  Port=6
  MGR_Out : Outport  Port=7
  wires:
  NOT/1 -> AND/2, AND2/2, AND3/2  "NRC_NOT_ACTIVE"
  Health Check/5(MGL_FLAGS) -> " Output Formatting"/5(MGL_FLAG)
  Health Check/2(MGL_FAIL) -> MGL_DSC_FAIL/1, AND1/2, AND2/1  "MGL_DSC_FAIL"
  Bus Selector/2 -> " Output Formatting"/14(MGL_WOW_Filt_N)  "<WOW_MGL_Filt_N>"
  Health Check/1(MGR_FAIL) -> MGR_DSC_FAIL/1, AND1/1, AND/1  "MGR_DSC_FAIL"
  Health Check/8(MGL_HEALTH) -> Bus Assignment1/1
  Health Check/4(MGR_FLAGS) -> " Output Formatting"/4(MGR_FLAG)
  Health Check/3(NG_FAIL) -> AND3/1, NG_DSC_FAIL/1  "NG_DSC_FAIL"
  Health Check/6(NG_FLAGS) -> " Output Formatting"/6(NG_FLAG)
  Bus Selector/3 -> " Output Formatting"/15(NG_WOW_Filt_N)  "<WOW_NG_Filt_N>"
  MGL FLAG Word/1 -> Health Check/4(MGL FLAG Word)
  NG STAT Word/1 -> Health Check/7(NG STAT Word)
  Health Check/9(NG_HEALTH) -> Bus Assignment2/1
  AND2/1 -> " Output Formatting"/2(MGL_RESET_REQUEST)  "RESET_REQUEST"
  Bus Selector/1 -> " Output Formatting"/13(MGR_WOW_Filt_N)  "<WOW_MGR_Filt_N>"
  AND/1 -> " Output Formatting"/1(MGR_RESET_REQUEST)  "RESET_REQUEST"
  NG FLAG Word/1 -> Health Check/6(NG FLAG Word)
  Health Check/7(MGR_HEALTH) -> Bus Assignment/1
  AND3/1 -> " Output Formatting"/3(NG_RESET_REQUEST)  "RESET_REQUEST"
  MGR FLAG Word/1 -> Health Check/2(MGR FLAG Word)
  WOW_Bus/1 -> Bus Selector/1, Health Check/14(WOW_N)
  MGR STAT Word/1 -> Health Check/3(MGR STAT Word)
  MGL STAT Word/1 -> Health Check/5(MGL STAT Word)
  NRC Active/1 -> NOT/1
  " Output Formatting"/2(MGL_Out) -> MGL_Out/1
  " Output Formatting"/3(MGR_Out) -> MGR_Out/1
  " Output Formatting"/1(NG_Out) -> NG_Out/1
  AND1/1 -> OUTPUT_DISABLE/1
  Health Check/10(MGR_STAT) -> " Output Formatting"/10(MGR_STAT)
  Health Check/11(MGL_STAT) -> " Output Formatting"/11(MGL_STAT)
  Health Check/12(NG_STAT) -> " Output Formatting"/12(NG_STAT)
  PIC_AP_MODE/1 -> Health Check/1(PIC_AP_MODE)
  MGR_STALE_LOAD/1 -> Comms Timeout Logic/1(MGR_STALE_LOAD)
  MGL_STALE_LOAD/1 -> Comms Timeout Logic/2(MGL_STALE_LOAD)
  NG_STALE_LOAD/1 -> Comms Timeout Logic/3(NG_STALE_LOAD)
  MGR_STALE_FLAGS/1 -> Comms Timeout Logic/4(MGR_STALE_FLAG)
  MGL_STALE_FLAGS/1 -> Comms Timeout Logic/5(MGL_STALE_FLAG)
  NG_STALE_FLAGS/1 -> Comms Timeout Logic/6(NG_STALE_FLAG)
  INIT/1 -> Comms Timeout Logic/7(INIT)
  Comms Timeout Logic/1(MGR_LOAD_TIMEOUT) -> Health Check/8(MGR_LOAD_TIMEOUT)
  Comms Timeout Logic/2(MGL_LOAD_TIMEOUT) -> Health Check/9(MGL_LOAD_TIMEOUT)
  Comms Timeout Logic/3(NG_LOAD_TIMEOUT) -> Health Check/10(NG_LOAD_TIMEOUT)
  Comms Timeout Logic/4(MGR_FLAG_TIMEOUT) -> Health Check/11(MGR_FLAG_TIMEOUT)
  Comms Timeout Logic/5(MGL_FLAG_TIMEOUT) -> Health Check/12(MGL_FLAG_TIMEOUT)
  Comms Timeout Logic/6(NG_FLAG_TIMEOUT) -> Health Check/13(NG_FLAG_TIMEOUT)
  Bus Assignment/1 -> " Output Formatting"/7(MGR_HEALTH)
  Bus Assignment1/1 -> " Output Formatting"/8(MGL_HEALTH)
  Bus Assignment2/1 -> " Output Formatting"/9(NG_HEALTH)
  Comms Timeout Logic/7(MGR_ACTIVE) -> AND/3, Bus Assignment/2
  Comms Timeout Logic/8(MGL_ACTIVE) -> AND2/3, Bus Assignment1/2
  Comms Timeout Logic/9(NG_ACTIVE) -> Bus Assignment2/2, AND3/3

== system Lib_Piccolo/Ground Detection Systems/WoW Wrapper/Variant Subsystem/Load Cell WoW Model 21/WOW Module/T//O Configuration ==
  note: Unlike when landing our persistance and latching is inverted relative to Weight Off both gears.
      |
      | Protection against WOW Failure. In the Event of a Sensor Failure and AC lift's off, NZ threshold overides WOW signal.
  PICCOLO_AP_MODE : Inport
  WOW_Filt : Inport  Port=2
  DSC_Fail : Inport  Port=3
  AND : Logic  IconShape=distinctive  AllPortsSameDT=off  OutDataTypeStr=boolean
  Bus Selector : BusSelector  OutputSignals=WOW_Filt_NG_N,WOW_Filt_MGL_N,WOW_Filt_MGR_N
  Bus Selector1 : BusSelector  OutputSignals=MGR_DSC_FAIL,MGL_DSC_FAIL
  Compare To Constant1 : simulink/Logic and Bit Operations/Compare To Constant  relop=<  const=SensorModel.WOW.Cell.TO_loadThreshold_N  OutDataTypeStr=uint8
  Compare To Constant2 : simulink/Logic and Bit Operations/Compare To Constant  relop=<  const=SensorModel.WOW.Cell.TO_loadThreshold_N  OutDataTypeStr=uint8
  Compare To Constant6 : simulink/Logic and Bit Operations/Compare To Constant  relop=>=  const=2  OutDataTypeStr=uint8
  Input Selection (Failure Handling) : $bdroot/Ground Detection Systems/WoW Wrapper/Variant Subsystem/Load Cell WoW Model 20/WOW Module/Landing Configuration/Input Selection (Failure Handling)  SystemSampleTime=-1
  Latch : Subsystem
  Latch Timer : Subsystem  mask{period=SensorModel.WOW.Cell.TO_latchTime_s}
      mask prompts: period "Period [s]"
  Latch Timer1 : $bdroot/Ground Detection Systems/WoW Wrapper/Variant Subsystem/Load Cell WoW Model 21/WOW Module/T//O Configuration/Latch Timer  period=SensorModel.WOW.Cell.TO_latchTime_s
  Latch1 : $bdroot/Ground Detection Systems/WoW Wrapper/Variant Subsystem/Load Cell WoW Model 21/WOW Module/T//O Configuration/Latch  SystemSampleTime=-1
  NOT : Logic  Operator=NOT  IconShape=distinctive  AllPortsSameDT=off  OutDataTypeStr=boolean
  NOT1 : Logic  Operator=NOT  IconShape=distinctive  AllPortsSameDT=off  OutDataTypeStr=boolean
  NOT3 : Logic  Operator=NOT  IconShape=distinctive  AllPortsSameDT=off  OutDataTypeStr=boolean
  OR : Logic  Operator=OR  IconShape=distinctive  AllPortsSameDT=off  OutDataTypeStr=boolean
  Persistance Timer : Subsystem  mask{period=SensorModel.WOW.Cell.TO_persistanceTime2_s}
      mask prompts: period "Period [s]"
  Persistance Timer1 : $bdroot/Ground Detection Systems/WoW Wrapper/Variant Subsystem/Load Cell WoW Model 21/WOW Module/T//O Configuration/Persistance Timer  period=SensorModel.WOW.Cell.TO_persistanceTime_s
  Terminator : Terminator
  Unit Delay : UnitDelay  SampleTime=-1
  Unit Delay1 : UnitDelay  SampleTime=-1
  ContactBool : Outport
  Takeoff_Fail_L : Outport  Port=2
  Takeoff_Fail_R : Outport  Port=3
  wires:
  Persistance Timer/1(Expired) -> Latch/1(D)
  Compare To Constant2/1 -> AND/1
  Latch Timer/1(Expired) -> NOT/1
  Unit Delay/1 -> Latch Timer/1(Enable/!Rst)
  Compare To Constant1/1 -> AND/2
  Latch/1(Q_Latched) -> Unit Delay/1, OR/1  "ContactBool"
  NOT/1 -> Latch/2(Enable/!Rst)
  WOW_Filt/1 -> Bus Selector/1
  Bus Selector/1 -> Terminator/1  "<WOW_Filt_NG_N>"
  Bus Selector/2 -> Input Selection (Failure Handling)/1  "<WOW_Filt_MGL_N>"
  Bus Selector/3 -> Input Selection (Failure Handling)/2  "<WOW_Filt_MGR_N>"
  DSC_Fail/1 -> Bus Selector1/1
  Bus Selector1/1 -> Input Selection (Failure Handling)/3  "<MGR_DSC_FAIL>"
  Bus Selector1/2 -> Input Selection (Failure Handling)/4  "<MGL_DSC_FAIL>"
  Input Selection (Failure Handling)/1 -> Compare To Constant2/1  "InputL"
  Input Selection (Failure Handling)/2 -> Compare To Constant1/1  "InputR"
  Input Selection (Failure Handling)/3 -> Takeoff_Fail_L/1
  Input Selection (Failure Handling)/4 -> Takeoff_Fail_R/1
  PICCOLO_AP_MODE/1 -> Compare To Constant6/1
  Compare To Constant6/1 -> Persistance Timer/1(Enable/!Rst)
  NOT1/1 -> Latch1/2
  AND/1 -> Persistance Timer1/1
  Unit Delay1/1 -> Latch Timer1/1
  Latch Timer1/1 -> NOT1/1
  Latch1/1 -> OR/2, Unit Delay1/1  "ContactBool"
  Persistance Timer1/1 -> Latch1/1
  OR/1 -> NOT3/1
  NOT3/1 -> ContactBool/1
